simulink model "Aufgabe2c"  (R2020a)
settings: Solver=VariableStepAuto  StartTime=0.0  StopTime=10.0  RelTol=1e-3
undefined symbols (not defined in the file or in its folder): A, B, C, D, J, psi, r, R, x0
settings Model: Creator=Ravi Plenzdorf  LastModifiedBy=Ravi Plenzdorf
settings DataIOCC: ReturnWorkspaceOutputs=off

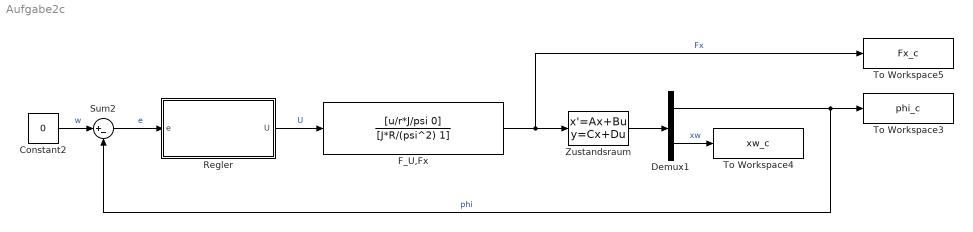
== system Aufgabe2c ==
  Constant2 : Constant  Value=0
  Demux1 : Demux  Outputs=2
  F_U,Fx : TransferFcn  Numerator=[u/r*J/psi 0]  Denominator=[J*R/(psi^2) 1]
  Regler : Subsystem
  Sum2 : Sum  Inputs=|+-
  To Workspace3 : ToWorkspace  VariableName=phi_c  SaveFormat=Timeseries  SampleTime=-1
  To Workspace4 : ToWorkspace  VariableName=xw_c  SaveFormat=Timeseries  SampleTime=-1
  To Workspace5 : ToWorkspace  VariableName=Fx_c  SaveFormat=Timeseries  SampleTime=-1
  Zustandsraum : StateSpace  A=A  B=B  C=C  D=D  InitialCondition=x0
  wires:
  Zustandsraum/1 -> Demux1/1
  Sum2/1 -> Regler/1(e)  "e"
  Regler/1(U) -> F_U,Fx/1  "U"
  Demux1/2 -> To Workspace4/1  "xw"
  Demux1/1 -> Sum2/2, To Workspace3/1  "phi"
  Constant2/1 -> Sum2/1  "w"
  F_U,Fx/1 -> Zustandsraum/1, To Workspace5/1  "Fx"

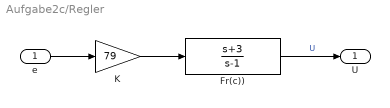
== system Aufgabe2c/Regler ==
  e : Inport
  Fr(c)) : TransferFcn  Numerator=[1 +3]  Denominator=[1 -1]
  K : Gain  Gain=79
  U : Outport
  wires:
  Fr(c))/1 -> U/1  "U"
  K/1 -> Fr(c))/1
  e/1 -> K/1
